simulink model "prac_Lab_04b"  (R2024b)
settings: Solver=VariableStepAuto  StartTime=0.0  StopTime=10.0  RelTol=1e-3
undefined symbols (not defined in the file or in its folder): Angle, Magnitude
libraries: spsCurrentMeasurementLib x3, spsLinearTransformerLib x2, spsSeriesRLCBranchLib x2, spsACVoltageSourceLib x1, spsVoltageMeasurementLib x1, sps_lib x1

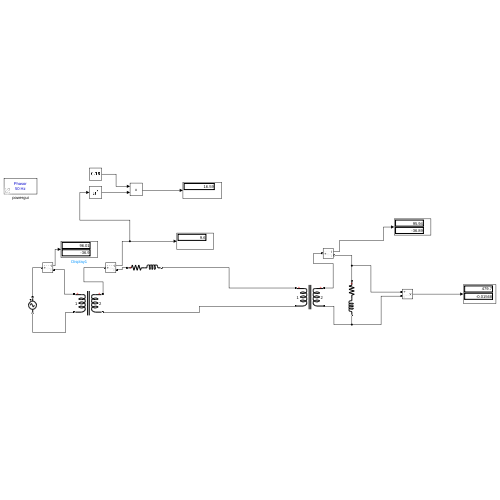
[thumbnail: Simulink's stored preview of the top-level diagram]
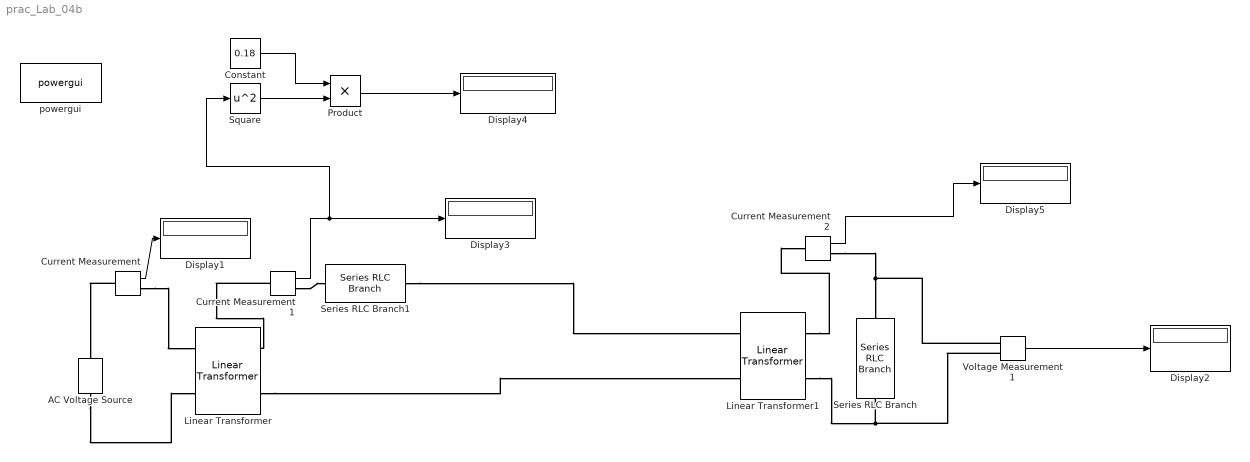
== system prac_Lab_04b ==
  AC Voltage Source : spsACVoltageSourceLib/AC Voltage Source  Amplitude=480  Phase=0  Frequency=50  SampleTime=0  Measurements=None  BusType=swing  Pref=10e3  Qref=0  Qmin=-inf  Qmax=+inf
  Constant : Constant  Value=0.18
  Current Measurement : spsCurrentMeasurementLib/Current Measurement  PhasorSimulation=on  OutputType=Magnitude-Angle  PSBequivalent=0
  Current Measurement1 : spsCurrentMeasurementLib/Current Measurement  PhasorSimulation=on  OutputType=Magnitude  PSBequivalent=0
  Current Measurement2 : spsCurrentMeasurementLib/Current Measurement  PhasorSimulation=on  OutputType=Magnitude-Angle  PSBequivalent=0
  Display{1..5} (5 alike) : Display
      Display4 settings: Format=bank
  Linear Transformer : spsLinearTransformerLib/Linear Transformer  UNITS=SI  NominalPower=[ 250e6 50 ]  winding1=[480 0.000001 0.000001]  winding2=[4800 0.000001 0.00001]  ThreeWindings=off  winding3=[3.15e+05 0.7938 0.084225]  RmLm=[1.0804e+06 2866]  Measurements=None  DataType=on
  Linear Transformer1 : spsLinearTransformerLib/Linear Transformer  UNITS=SI  NominalPower=[ 250e6 50 ]  winding1=[4800 0.00001 0.000001]  winding2=[480 0.000001 0.000001]  ThreeWindings=off  winding3=[3.15e+05 0.7938 0.084225]  RmLm=[1.0804e+06 2866]  Measurements=None  DataType=on
  Product : Product
  Series RLC Branch : spsSeriesRLCBranchLib/Series RLC Branch  LConnTagsString=__new0  RConnTagsString=__new0  BranchType=RL  Resistance=4  Inductance=3/(2*pi*50)  SetiL0=off  InitialCurrent=0  Capacitance=1e-6  Setx0=off  InitialVoltage=0  Measurements=None
  Series RLC Branch1 : spsSeriesRLCBranchLib/Series RLC Branch  LConnTagsString=__new0  RConnTagsString=__new0  BranchType=RL  Resistance=0.18  Inductance=0.24/(2*pi*50)  SetiL0=off  InitialCurrent=0  Capacitance=1e-6  Setx0=off  InitialVoltage=0  Measurements=None
  Square : Math  Operator=square
  Voltage Measurement1 : spsVoltageMeasurementLib/Voltage Measurement  PhasorSimulation=on  OutputType=Magnitude-Angle  PSBequivalent=0
  powergui : sps_lib/powergui  Priority=1  SimulationMode=Phasor  SampleTime=50e-6  frequency=50  Iterations=50  frequencyindice=50  Pbase=100e6  ErrMax=1e-4  UnitsV=kV  UnitsW=MW  buscounter=0  FunctionMessages=off  echomessages=off  EnableUseOfTLC=off  CurrentSourceSwitches=off  DisableSnubberDevices=off  DisableRonSwitches=off  DisableVfSwitches=off  DisplayEquations=off  AutomaticDiscreteSolvers=off  SolverType=Tustin/Backward Euler (TBE)  Interpol=off  ExternalGateDelay=off  methode=off  Ts=100  x0status=blocks  SPID=on  SwTol=0  HookPort=off  NonlinearTolerance=1e-4  nMaxIteration=100  ContinueOnMaxIteration=off  RestoreLinks=warning  ResistiveCurrentMeasurement=off  Frange=[0:2:500]  Ylog=off  Xlog=on  ShowGrid=off  save=off  variable=ZData  structure=0  ZoomFFT=off  StartTime=0.0  cycles=1  DisplayStyle=1  fundamental=60  FreqAxis=off  MaxFrequency=1000  frequencyindicesteady=1  RmsSteady=1  display=off
  wires:
  Constant/1 -> Product/1
  Product/1 -> Display4/1
  Voltage Measurement1/1 -> Display2/1
  Square/1 -> Product/2
  Current Measurement1/1 -> Square/1, Display3/1
  Current Measurement2/1 -> Display5/1
  Current Measurement/1 -> Display1/1
  connections:
  Voltage Measurement1/LConn1 -- Current Measurement2/RConn1 -- Series RLC Branch/LConn1
  AC Voltage Source/LConn1 -- Linear Transformer/LConn2
  Current Measurement/LConn1 -- AC Voltage Source/RConn1
  Current Measurement/RConn1 -- Linear Transformer/LConn1
  Current Measurement1/LConn1 -- Linear Transformer/RConn1
  Current Measurement1/RConn1 -- Series RLC Branch1/LConn1
  Series RLC Branch1/RConn1 -- Linear Transformer1/LConn1
  Linear Transformer/RConn2 -- Linear Transformer1/LConn2
  Linear Transformer1/RConn2 -- Voltage Measurement1/LConn2 -- Series RLC Branch/RConn1
  Linear Transformer1/RConn1 -- Current Measurement2/LConn1
